simulink model "engine"  (R2024b)
settings: Solver=ode113  StartTime=0.0  StopTime=7  FixedStep=0.01  RelTol=1e-5  AbsTol=1e-7
undefined symbols (not defined in the file): ENG
settings Model: Creator=Leonardo Perina  LastModifiedBy=Leonardo Perina

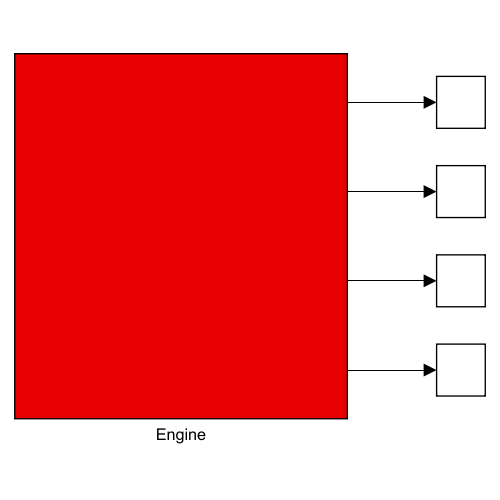
[thumbnail: Simulink's stored preview of the top-level diagram]
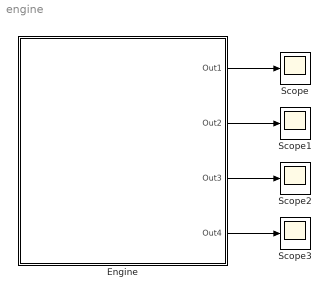
== system engine ==
  Engine : Subsystem
  Scope{,1..3} (4 alike) : Scope
  wires:
  Engine/1(Out1) -> Scope/1
  Engine/2(Out2) -> Scope1/1
  Engine/3(Out3) -> Scope2/1
  Engine/4(Out4) -> Scope3/1

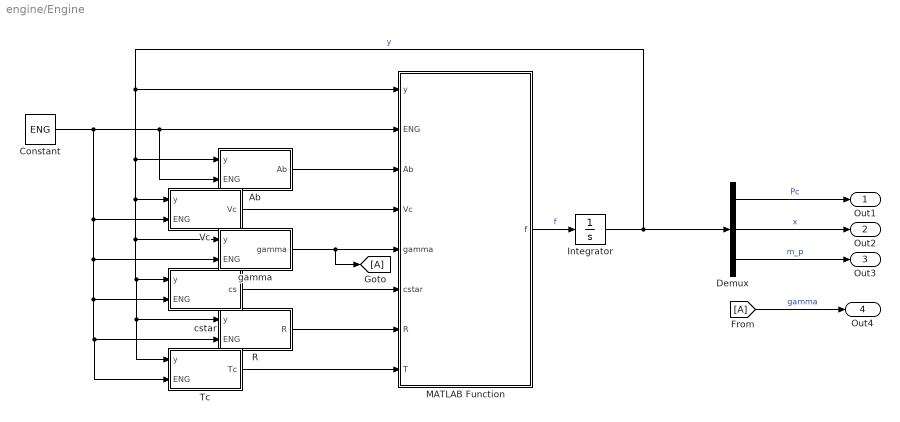
== system engine/Engine ==
  Ab : MATLAB Function  TreatAsAtomicUnit=on
  Constant : Constant  Value=ENG  OutDataTypeStr=Bus: ENGbus
  Demux : Demux  Outputs=3
  From : From
  Goto : Goto
  Integrator : Integrator  InitialCondition=ENG.y0
  MATLAB Function : MATLAB Function  TreatAsAtomicUnit=on
  R : MATLAB Function  TreatAsAtomicUnit=on
  Tc : MATLAB Function  TreatAsAtomicUnit=on
  Vc : MATLAB Function  TreatAsAtomicUnit=on
  cstar : MATLAB Function  TreatAsAtomicUnit=on
  gamma : MATLAB Function  TreatAsAtomicUnit=on
  Out1 : Outport
  Out2 : Outport  Port=2
  Out3 : Outport  Port=3
  Out4 : Outport  Port=4
  wires:
  MATLAB Function/1(f) -> Integrator/1  "f"
  Integrator/1 -> Demux/1, MATLAB Function/1(y), Ab/1(y), Tc/1(y), R/1(y), cstar/1(y), gamma/1(y), Vc/1(y)  "y"
  Constant/1 -> Tc/2(ENG), R/2(ENG), cstar/2(ENG), gamma/2(ENG), Vc/2(ENG), Ab/2(ENG), MATLAB Function/2(ENG)
  Ab/1(Ab) -> MATLAB Function/3(Ab)
  Vc/1(Vc) -> MATLAB Function/4(Vc)
  gamma/1(gamma) -> Goto/1, MATLAB Function/5(gamma)
  cstar/1(cs) -> MATLAB Function/6(cstar)
  Tc/1(Tc) -> MATLAB Function/8(T)
  R/1(R) -> MATLAB Function/7(R)
  Demux/1 -> Out1/1  "Pc"
  Demux/2 -> Out2/1  "x"
  Demux/3 -> Out3/1  "m_p"
  From/1 -> Out4/1  "gamma"

== matlab function engine/Engine/Ab ==
  data: y input; Ab output; ENG input
function Ab = fcn(y, ENG)

x = y(2);

Ab = interp1(ENG.grain(:, 3), ENG.grain(:, 1), x);

== matlab function engine/Engine/MATLAB Function ==
  data: f output; y input; ENG input; Ab input; Vc input; gamma input; cstar input; R input; T input
function f  = internal_balistics(y, ENG, Ab, Vc, gamma, cstar, R, T)
%INTERNAL_BALISTICS function determining the internal balistics of the
% rocket engine. 
% The elements of the state space vector are: chamber pressure, grain
% regression, m_propellant_exited

% Pc = max(y(1), 1e4);                                                      % Pa
Pc = y(1);
x  = y(2);                                                                  % m

%_______________________________________________________________ grain data
if x < ENG.xfin
    rb = ENG.a * Pc.^ENG.n;
else
    Ab = 0;
    rb = 0;
    f  = zeros(3, 1);
    return
end

%__________________________________________________________ propellant data
Pcbar = Pc / 1e5;
if Pcbar > max(ENG.Pbar) * 2
    warning('Pressure is over double the maximum tabulated pressure')
    fprintf('Pc [bar] at the moment: %f bar\n', Pcbar)
    fprintf('Maximum tabulated pressure: %f bar\n', max(ENG.Pbar))
    warning('Warning! There is also the possibility that this is a rejected step by the ode() function')
end

PR = min(101325 / Pc, 0.999);
choked = 1/PR > ( (gamma + 1)/2 )^(gamma/(gamma-1));

if choked
    % cstar = ENGfnc.cs(Pcbar);
    mdot  = Pc * ENG.At / cstar;
else

    
    mdot = ENG.At * Pc * sqrt(gamma/(R*T)) * ...
           PR^(1/gamma) * ...
           sqrt(2/(gamma-1) * (1 - PR^((gamma-1)/gamma)));
end



mdot_gen = ENG.rhop * rb * Ab;
Rt = R * T;

f = zeros(3, 1);


f(1) = Rt / Vc * (mdot_gen - mdot);
f(2) = rb;
f(3) = -mdot;
end

== matlab function engine/Engine/Vc ==
  data: y input; Vc output; ENG input
function Vc = fcn(y, ENG)

x = y(2);

Vc = interp1(ENG.grain(:, 3), ENG.grain(:, 2), x).*ENG.L;

== matlab function engine/Engine/gamma ==
  data: y input; gamma output; ENG input
function gamma = fcn(y, ENG)

P = y(1) / 1e5;

gamma = interp1(ENG.Pbar, ENG.propl(:, 3), P);

== matlab function engine/Engine/cstar ==
  data: y input; cs output; ENG input
function cs = fcn(y, ENG)

P = y(1) / 1e5;

cs = interp1(ENG.Pbar, ENG.propl(:, 6), P);

== matlab function engine/Engine/R ==
  data: y input; R output; ENG input
function R = fcn(y, ENG)

P = y(1) / 1e5;

R = interp1(ENG.Pbar, ENG.propl(:, 5), P);

== matlab function engine/Engine/Tc ==
  data: y input; Tc output; ENG input
function Tc = fcn(y, ENG)

P = y(1) / 1e5;

Tc = interp1(ENG.Pbar, ENG.propl(:, 2), P);
